simulink model "Task_8"  (R2022b)
settings: Solver=VariableStepAuto  StartTime=0.0  StopTime=10.0  RelTol=1e-3
settings Model: Creator=Abanob_Sameh  LastModifiedBy=Abanob_Sameh

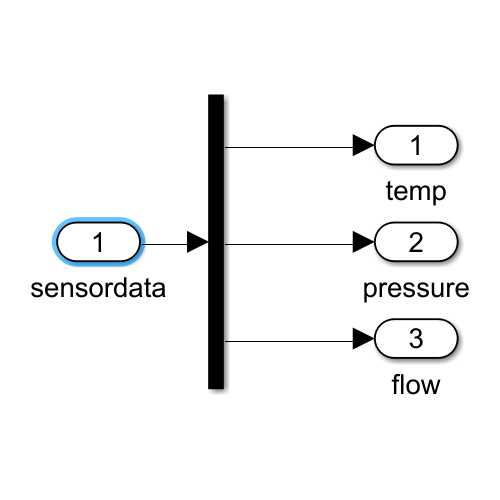
[thumbnail: Simulink's stored preview of the top-level diagram]
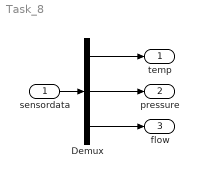
== system Task_8 ==
  sensordata : Inport
  Demux : Demux  Outputs=3
  temp : Outport
  pressure : Outport  Port=2
  flow : Outport  Port=3
  wires:
  Demux/3 -> flow/1
  sensordata/1 -> Demux/1
  Demux/1 -> temp/1
  Demux/2 -> pressure/1
